simulink model "VehicleBody6DOFSSC"  (R2026b)
settings: Solver=VariableStepAuto
undefined symbols (not defined in the file): EnvAirDen, PlntVehAeroDragCff, PlntVehAeroFrntArea, PlntVehAeroLiftCff, PlntVehCGHgtAxl, PlntVehDstCGFrntAxl, PlntVehDstCGRearAxl, PlntVehInitLatPos, PlntVehInitVertPos, PlntVehMass, PlntVehMultiBody, PlntVehPitchMomentInertia, PlntVehRollMomentInertia, PlntVehTrckWdth, PlntVehYawMomentInertia, X, Y, Z
libraries: nesl_utility x68, sm_lib x60, sharedtransform x22, fl_lib x6, vehdynlibeomcommon x1, autolibutils x1
(part 3 of 3)

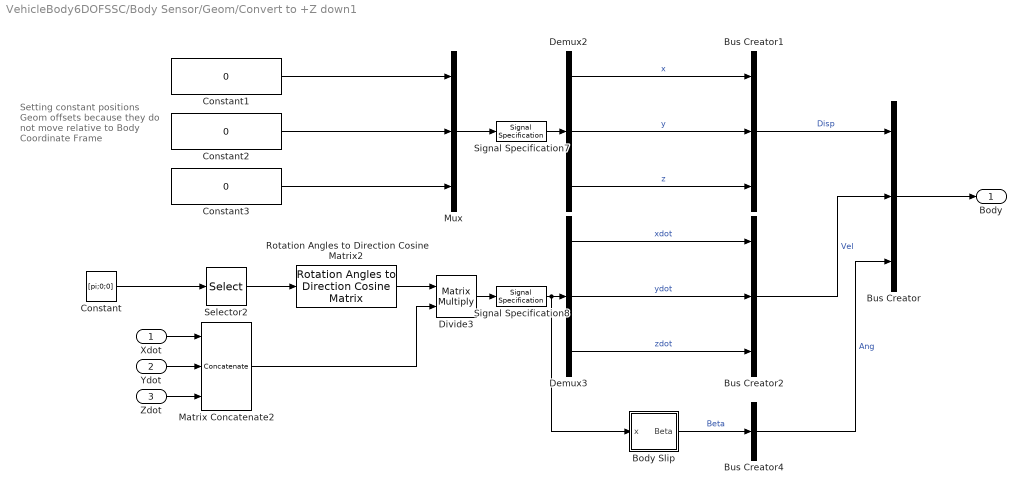
== system VehicleBody6DOFSSC/Body Sensor/Geom/Convert to +Z down1 ==
  note: Setting constant
      | positions Geom offsets
      | because they do not
      | move relative to Body
      | Coordinate Frame
  Xdot : Inport
  Ydot : Inport  Port=2
  Zdot : Inport  Port=3
  Body Slip : Subsystem
  Bus Creator : BusCreator  Inputs=3
  Bus Creator1 : BusCreator  Inputs=3
  Bus Creator2 : BusCreator  Inputs=3
  Bus Creator4 : BusCreator  Inputs=1
  Constant : Constant  Value=[pi;0;0]  SampleTime=-1
  Constant1 : Constant  Value=0  SampleTime=-1
  Constant2 : Constant  Value=0  SampleTime=-1
  Constant3 : Constant  Value=0  SampleTime=-1
  Demux2 : Demux  Outputs=3
  Demux3 : Demux  Outputs=3
  Divide3 : Product  Inputs=**  Multiplication=Matrix(*)
  Matrix Concatenate2 : Concatenate  NumInputs=3  Mode=Multidimensional array
  Mux : Mux  Inputs=3
  Rotation Angles to Direction Cosine Matrix2 : sharedtransform/Rotation Angles to Direction Cosine Matrix  rotationOrder=ZYX  aMode=2
  Selector2 : Selector  InputPortWidth=3  IndexOptions=Index vector (dialog)  Indices=[3 2 1]  OutputSizes=1
  Signal Specification7 : SignalSpecification  Unit=m
  Signal Specification8 : SignalSpecification  Unit=m/s
  Body : Outport
  wires:
  Bus Creator4/1 -> Bus Creator/3  "Ang"
  Signal Specification8/1 -> Demux3/1, Body Slip/1(x)
  Body Slip/1(Beta) -> Bus Creator4/1  "Beta"
  Bus Creator1/1 -> Bus Creator/1  "Disp"
  Bus Creator/1 -> Body/1
  Bus Creator2/1 -> Bus Creator/2  "Vel"
  Constant3/1 -> Mux/3
  Constant1/1 -> Mux/1
  Constant2/1 -> Mux/2
  Mux/1 -> Signal Specification7/1
  Signal Specification7/1 -> Demux2/1
  Demux2/2 -> Bus Creator1/2  "y"
  Demux3/3 -> Bus Creator2/3  "zdot"
  Demux2/3 -> Bus Creator1/3  "z"
  Demux3/2 -> Bus Creator2/2  "ydot"
  Demux3/1 -> Bus Creator2/1  "xdot"
  Demux2/1 -> Bus Creator1/1  "x"
  Zdot/1 -> Matrix Concatenate2/3
  Ydot/1 -> Matrix Concatenate2/2
  Selector2/1 -> Rotation Angles to Direction Cosine Matrix2/1
  Rotation Angles to Direction Cosine Matrix2/1 -> Divide3/1
  Constant/1 -> Selector2/1
  Xdot/1 -> Matrix Concatenate2/1
  Matrix Concatenate2/1 -> Divide3/2
  Divide3/1 -> Signal Specification8/1

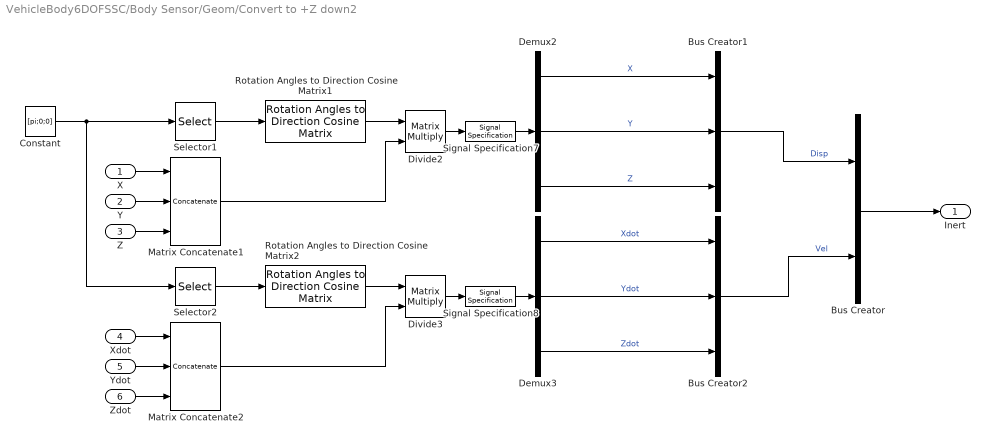
== system VehicleBody6DOFSSC/Body Sensor/Geom/Convert to +Z down2 ==
  X : Inport
  Y : Inport  Port=2
  Z : Inport  Port=3
  Xdot : Inport  Port=4
  Ydot : Inport  Port=5
  Zdot : Inport  Port=6
  Bus Creator : BusCreator  Inputs=2
  Bus Creator1 : BusCreator  Inputs=3
  Bus Creator2 : BusCreator  Inputs=3
  Constant : Constant  Value=[pi;0;0]  SampleTime=-1
  Demux2 : Demux  Outputs=3
  Demux3 : Demux  Outputs=3
  Divide2 : Product  Inputs=**  Multiplication=Matrix(*)
  Divide3 : Product  Inputs=**  Multiplication=Matrix(*)
  Matrix Concatenate1 : Concatenate  NumInputs=3  Mode=Multidimensional array
  Matrix Concatenate2 : Concatenate  NumInputs=3  Mode=Multidimensional array
  Rotation Angles to Direction Cosine Matrix1 : sharedtransform/Rotation Angles to Direction Cosine Matrix  rotationOrder=ZYX  aMode=2
  Rotation Angles to Direction Cosine Matrix2 : sharedtransform/Rotation Angles to Direction Cosine Matrix  rotationOrder=ZYX  aMode=2
  Selector1 : Selector  InputPortWidth=3  IndexOptions=Index vector (dialog)  Indices=[3 2 1]  OutputSizes=1
  Selector2 : Selector  InputPortWidth=3  IndexOptions=Index vector (dialog)  Indices=[3 2 1]  OutputSizes=1
  Signal Specification7 : SignalSpecification  Unit=m
  Signal Specification8 : SignalSpecification  Unit=m/s
  Inert : Outport
  wires:
  Bus Creator/1 -> Inert/1
  Bus Creator2/1 -> Bus Creator/2  "Vel"
  Bus Creator1/1 -> Bus Creator/1  "Disp"
  Divide3/1 -> Signal Specification8/1
  Matrix Concatenate2/1 -> Divide3/2
  Xdot/1 -> Matrix Concatenate2/1
  Constant/1 -> Selector1/1, Selector2/1
  Rotation Angles to Direction Cosine Matrix2/1 -> Divide3/1
  Selector2/1 -> Rotation Angles to Direction Cosine Matrix2/1
  Ydot/1 -> Matrix Concatenate2/2
  Zdot/1 -> Matrix Concatenate2/3
  Z/1 -> Matrix Concatenate1/3
  Y/1 -> Matrix Concatenate1/2
  Divide2/1 -> Signal Specification7/1
  Selector1/1 -> Rotation Angles to Direction Cosine Matrix1/1
  Rotation Angles to Direction Cosine Matrix1/1 -> Divide2/1
  X/1 -> Matrix Concatenate1/1
  Matrix Concatenate1/1 -> Divide2/2
  Demux2/1 -> Bus Creator1/1  "X"
  Demux3/1 -> Bus Creator2/1  "Xdot"
  Demux3/2 -> Bus Creator2/2  "Ydot"
  Demux2/3 -> Bus Creator1/3  "Z"
  Demux3/3 -> Bus Creator2/3  "Zdot"
  Demux2/2 -> Bus Creator1/2  "Y"
  Signal Specification7/1 -> Demux2/1
  Signal Specification8/1 -> Demux3/1

== system VehicleBody6DOFSSC/Body Sensor/RLAxle/Convert to +Z down1 ==
  note: Setting constant
      | positions for Body Disp
      | because they do not
      | move relative to Body
      | Coordinate Frame
  Xdot : Inport
  Ydot : Inport  Port=2
  Zdot : Inport  Port=3
  Bus Creator : BusCreator  Inputs=2
  Bus Creator1 : BusCreator  Inputs=3
  Bus Creator2 : BusCreator  Inputs=3
  Constant : Constant  Value=[pi;0;0]  SampleTime=-1
  Constant1 : Constant  Value=-PlntVehDstCGRearAxl  SampleTime=-1
  Constant2 : Constant  Value=-PlntVehTrckWdth(2)/2  SampleTime=-1
  Constant3 : Constant  Value=PlntVehCGHgtAxl  SampleTime=-1
  Demux2 : Demux  Outputs=3
  Demux3 : Demux  Outputs=3
  Divide3 : Product  Inputs=**  Multiplication=Matrix(*)
  Matrix Concatenate2 : Concatenate  NumInputs=3  Mode=Multidimensional array
  Mux : Mux  Inputs=3
  Rotation Angles to Direction Cosine Matrix2 : sharedtransform/Rotation Angles to Direction Cosine Matrix  rotationOrder=ZYX  aMode=2
  Selector2 : Selector  InputPortWidth=3  IndexOptions=Index vector (dialog)  Indices=[3 2 1]  OutputSizes=1
  Signal Specification7 : SignalSpecification  Unit=m
  Signal Specification8 : SignalSpecification  Unit=m/s
  Body : Outport
  wires:
  Bus Creator1/1 -> Bus Creator/1  "Disp"
  Bus Creator/1 -> Body/1
  Bus Creator2/1 -> Bus Creator/2  "Vel"
  Constant3/1 -> Mux/3
  Constant1/1 -> Mux/1
  Constant2/1 -> Mux/2
  Mux/1 -> Signal Specification7/1
  Signal Specification8/1 -> Demux3/1
  Signal Specification7/1 -> Demux2/1
  Demux2/2 -> Bus Creator1/2  "y"
  Demux3/3 -> Bus Creator2/3  "zdot"
  Demux2/3 -> Bus Creator1/3  "z"
  Demux3/2 -> Bus Creator2/2  "ydot"
  Demux3/1 -> Bus Creator2/1  "xdot"
  Demux2/1 -> Bus Creator1/1  "x"
  Zdot/1 -> Matrix Concatenate2/3
  Ydot/1 -> Matrix Concatenate2/2
  Selector2/1 -> Rotation Angles to Direction Cosine Matrix2/1
  Rotation Angles to Direction Cosine Matrix2/1 -> Divide3/1
  Constant/1 -> Selector2/1
  Xdot/1 -> Matrix Concatenate2/1
  Matrix Concatenate2/1 -> Divide3/2
  Divide3/1 -> Signal Specification8/1

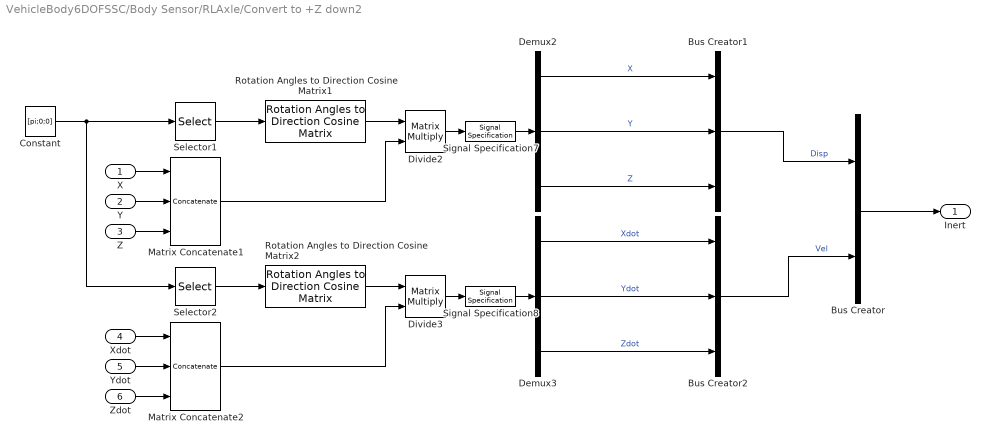
== system VehicleBody6DOFSSC/Body Sensor/RLAxle/Convert to +Z down2 ==
  X : Inport
  Y : Inport  Port=2
  Z : Inport  Port=3
  Xdot : Inport  Port=4
  Ydot : Inport  Port=5
  Zdot : Inport  Port=6
  Bus Creator : BusCreator  Inputs=2
  Bus Creator1 : BusCreator  Inputs=3
  Bus Creator2 : BusCreator  Inputs=3
  Constant : Constant  Value=[pi;0;0]  SampleTime=-1
  Demux2 : Demux  Outputs=3
  Demux3 : Demux  Outputs=3
  Divide2 : Product  Inputs=**  Multiplication=Matrix(*)
  Divide3 : Product  Inputs=**  Multiplication=Matrix(*)
  Matrix Concatenate1 : Concatenate  NumInputs=3  Mode=Multidimensional array
  Matrix Concatenate2 : Concatenate  NumInputs=3  Mode=Multidimensional array
  Rotation Angles to Direction Cosine Matrix1 : sharedtransform/Rotation Angles to Direction Cosine Matrix  rotationOrder=ZYX  aMode=2
  Rotation Angles to Direction Cosine Matrix2 : sharedtransform/Rotation Angles to Direction Cosine Matrix  rotationOrder=ZYX  aMode=2
  Selector1 : Selector  InputPortWidth=3  IndexOptions=Index vector (dialog)  Indices=[3 2 1]  OutputSizes=1
  Selector2 : Selector  InputPortWidth=3  IndexOptions=Index vector (dialog)  Indices=[3 2 1]  OutputSizes=1
  Signal Specification7 : SignalSpecification  Unit=m
  Signal Specification8 : SignalSpecification  Unit=m/s
  Inert : Outport
  wires:
  Bus Creator/1 -> Inert/1
  Bus Creator2/1 -> Bus Creator/2  "Vel"
  Bus Creator1/1 -> Bus Creator/1  "Disp"
  Divide3/1 -> Signal Specification8/1
  Matrix Concatenate2/1 -> Divide3/2
  Xdot/1 -> Matrix Concatenate2/1
  Constant/1 -> Selector1/1, Selector2/1
  Rotation Angles to Direction Cosine Matrix2/1 -> Divide3/1
  Selector2/1 -> Rotation Angles to Direction Cosine Matrix2/1
  Ydot/1 -> Matrix Concatenate2/2
  Zdot/1 -> Matrix Concatenate2/3
  Z/1 -> Matrix Concatenate1/3
  Y/1 -> Matrix Concatenate1/2
  Divide2/1 -> Signal Specification7/1
  Selector1/1 -> Rotation Angles to Direction Cosine Matrix1/1
  Rotation Angles to Direction Cosine Matrix1/1 -> Divide2/1
  X/1 -> Matrix Concatenate1/1
  Matrix Concatenate1/1 -> Divide2/2
  Demux2/1 -> Bus Creator1/1  "X"
  Demux3/1 -> Bus Creator2/1  "Xdot"
  Demux3/2 -> Bus Creator2/2  "Ydot"
  Demux2/3 -> Bus Creator1/3  "Z"
  Demux3/3 -> Bus Creator2/3  "Zdot"
  Demux2/2 -> Bus Creator1/2  "Y"
  Signal Specification7/1 -> Demux2/1
  Signal Specification8/1 -> Demux3/1

== system VehicleBody6DOFSSC/Body Sensor/RRAxle/Convert to +Z down1 ==
  note: Setting constant
      | positions for Body Disp
      | because they do not
      | move relative to Body
      | Coordinate Frame
  Xdot : Inport
  Ydot : Inport  Port=2
  Zdot : Inport  Port=3
  Bus Creator : BusCreator  Inputs=2
  Bus Creator1 : BusCreator  Inputs=3
  Bus Creator2 : BusCreator  Inputs=3
  Constant : Constant  Value=[pi;0;0]  SampleTime=-1
  Constant1 : Constant  Value=-PlntVehDstCGRearAxl  SampleTime=-1
  Constant2 : Constant  Value=PlntVehTrckWdth(2)/2  SampleTime=-1
  Constant3 : Constant  Value=PlntVehCGHgtAxl  SampleTime=-1
  Demux2 : Demux  Outputs=3
  Demux3 : Demux  Outputs=3
  Divide3 : Product  Inputs=**  Multiplication=Matrix(*)
  Matrix Concatenate2 : Concatenate  NumInputs=3  Mode=Multidimensional array
  Mux : Mux  Inputs=3
  Rotation Angles to Direction Cosine Matrix2 : sharedtransform/Rotation Angles to Direction Cosine Matrix  rotationOrder=ZYX  aMode=2
  Selector2 : Selector  InputPortWidth=3  IndexOptions=Index vector (dialog)  Indices=[3 2 1]  OutputSizes=1
  Signal Specification7 : SignalSpecification  Unit=m
  Signal Specification8 : SignalSpecification  Unit=m/s
  Body : Outport
  wires:
  Divide3/1 -> Signal Specification8/1
  Matrix Concatenate2/1 -> Divide3/2
  Xdot/1 -> Matrix Concatenate2/1
  Constant/1 -> Selector2/1
  Rotation Angles to Direction Cosine Matrix2/1 -> Divide3/1
  Selector2/1 -> Rotation Angles to Direction Cosine Matrix2/1
  Ydot/1 -> Matrix Concatenate2/2
  Zdot/1 -> Matrix Concatenate2/3
  Demux2/1 -> Bus Creator1/1  "x"
  Demux3/1 -> Bus Creator2/1  "xdot"
  Demux3/2 -> Bus Creator2/2  "ydot"
  Demux2/3 -> Bus Creator1/3  "z"
  Demux3/3 -> Bus Creator2/3  "zdot"
  Demux2/2 -> Bus Creator1/2  "y"
  Signal Specification7/1 -> Demux2/1
  Signal Specification8/1 -> Demux3/1
  Mux/1 -> Signal Specification7/1
  Constant2/1 -> Mux/2
  Constant1/1 -> Mux/1
  Constant3/1 -> Mux/3
  Bus Creator2/1 -> Bus Creator/2  "Vel"
  Bus Creator/1 -> Body/1
  Bus Creator1/1 -> Bus Creator/1  "Disp"

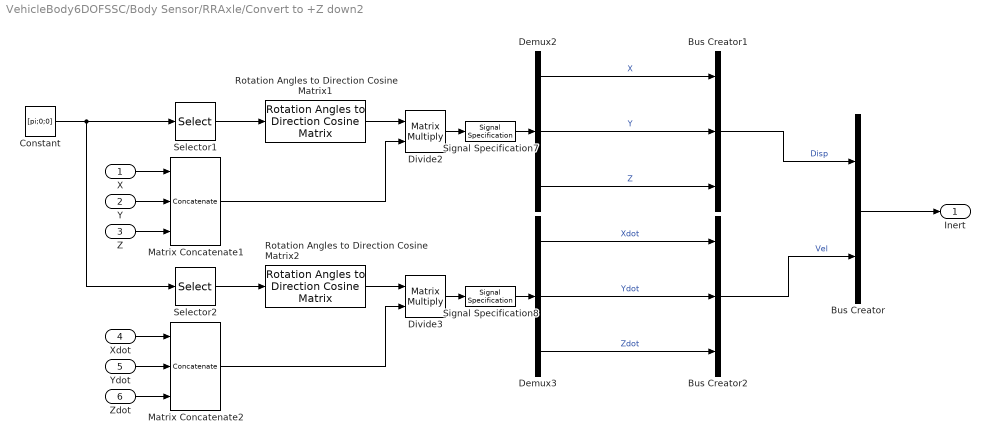
== system VehicleBody6DOFSSC/Body Sensor/RRAxle/Convert to +Z down2 ==
  X : Inport
  Y : Inport  Port=2
  Z : Inport  Port=3
  Xdot : Inport  Port=4
  Ydot : Inport  Port=5
  Zdot : Inport  Port=6
  Bus Creator : BusCreator  Inputs=2
  Bus Creator1 : BusCreator  Inputs=3
  Bus Creator2 : BusCreator  Inputs=3
  Constant : Constant  Value=[pi;0;0]  SampleTime=-1
  Demux2 : Demux  Outputs=3
  Demux3 : Demux  Outputs=3
  Divide2 : Product  Inputs=**  Multiplication=Matrix(*)
  Divide3 : Product  Inputs=**  Multiplication=Matrix(*)
  Matrix Concatenate1 : Concatenate  NumInputs=3  Mode=Multidimensional array
  Matrix Concatenate2 : Concatenate  NumInputs=3  Mode=Multidimensional array
  Rotation Angles to Direction Cosine Matrix1 : sharedtransform/Rotation Angles to Direction Cosine Matrix  rotationOrder=ZYX  aMode=2
  Rotation Angles to Direction Cosine Matrix2 : sharedtransform/Rotation Angles to Direction Cosine Matrix  rotationOrder=ZYX  aMode=2
  Selector1 : Selector  InputPortWidth=3  IndexOptions=Index vector (dialog)  Indices=[3 2 1]  OutputSizes=1
  Selector2 : Selector  InputPortWidth=3  IndexOptions=Index vector (dialog)  Indices=[3 2 1]  OutputSizes=1
  Signal Specification7 : SignalSpecification  Unit=m
  Signal Specification8 : SignalSpecification  Unit=m/s
  Inert : Outport
  wires:
  Signal Specification8/1 -> Demux3/1
  Signal Specification7/1 -> Demux2/1
  Demux2/2 -> Bus Creator1/2  "Y"
  Demux3/3 -> Bus Creator2/3  "Zdot"
  Demux2/3 -> Bus Creator1/3  "Z"
  Demux3/2 -> Bus Creator2/2  "Ydot"
  Demux3/1 -> Bus Creator2/1  "Xdot"
  Demux2/1 -> Bus Creator1/1  "X"
  Matrix Concatenate1/1 -> Divide2/2
  X/1 -> Matrix Concatenate1/1
  Rotation Angles to Direction Cosine Matrix1/1 -> Divide2/1
  Selector1/1 -> Rotation Angles to Direction Cosine Matrix1/1
  Divide2/1 -> Signal Specification7/1
  Y/1 -> Matrix Concatenate1/2
  Z/1 -> Matrix Concatenate1/3
  Zdot/1 -> Matrix Concatenate2/3
  Ydot/1 -> Matrix Concatenate2/2
  Selector2/1 -> Rotation Angles to Direction Cosine Matrix2/1
  Rotation Angles to Direction Cosine Matrix2/1 -> Divide3/1
  Constant/1 -> Selector2/1, Selector1/1
  Xdot/1 -> Matrix Concatenate2/1
  Matrix Concatenate2/1 -> Divide3/2
  Divide3/1 -> Signal Specification8/1
  Bus Creator1/1 -> Bus Creator/1  "Disp"
  Bus Creator2/1 -> Bus Creator/2  "Vel"
  Bus Creator/1 -> Inert/1

== system VehicleBody6DOFSSC/Body Sensor/Geom/Convert to +Z down1/Body Slip ==
  x : Inport
  Demux7 : Demux  Outputs=2
  Divide : Product  Inputs=*/
  Selector1 : Selector  IndexOptions=Index vector (dialog)  Indices=[2,1]  OutputSizes=1
  Signal Specification9 : SignalSpecification  Unit=rad
  Trigonometric Function : Trigonometry  Operator=atan  OutputSignalType=real
  div0protect - abs poly : autolibutils/div0protect - abs poly  thresh=eps  ZeroCross=off  aMode=2
  Beta : Outport  VectorParamsAs1DForOutWhenUnconnected=off
  wires:
  Demux7/2 -> div0protect - abs poly/1
  div0protect - abs poly/1 -> Divide/2
  Demux7/1 -> Divide/1
  x/1 -> Selector1/1
  Selector1/1 -> Demux7/1
  Trigonometric Function/1 -> Signal Specification9/1  "Beta"
  Divide/1 -> Trigonometric Function/1
  Signal Specification9/1 -> Beta/1
